simulink model "Synthgas"  (R2025a)
settings: Solver=VariableStepAuto  StartTime=0.0  StopTime=3600  RelTol=1e-3
PreLoadFcn:
  | run('params_wte.m');
  | run('PEMElectrolysisSystemParameters.m');
  | run('params_co2el.m');
InitFcn:
  | run(fullfile(fileparts(bdroot),'params_wte.m'));
  | run(fullfile(fileparts(bdroot),'PEMElectrolysisSystemParameters.m'));
  | run(fullfile(fileparts(bdroot),'params_co2el.m'));
values from neighbouring files (symbols this model uses):
  A = [ -1/tauQ,        0 ... (first row only)    [params_wte.m]
  A_cm2 = 200    [params_co2el.m]
  alpha = wC * eta_burn * (44/12)    (= 1.43733333333)    [params_wte.m]
  B = [ (eta_th*LHV)/(1e6*tauQ) ... (first row only)    [params_wte.m]
  C = [0, 1]    [params_wte.m]
  D = 0    [params_wte.m]
  env_T = 20    [PEMElectrolysisSystemParameters.m]
  exchanger_air_area_fins = 2 * exchanger_N_fins * exchanger_W * exchanger_gap_H    (= 11.5625)    [PEMElectrolysisSystemParameters.m]
  exchanger_air_area_primary = 2 * (exchanger_N_tubes - 1) * exchanger_W * (exchanger_L + exchanger_gap_H)    (= 1.223125)    [PEMElectrolysisSystemParameters.m]
  exchanger_eta_fin = 0.7    [PEMElectrolysisSystemParameters.m]
  exchanger_N_tubes = 25    [PEMElectrolysisSystemParameters.m]
  exchanger_tube_H = 0.0015    [PEMElectrolysisSystemParameters.m]
  exchanger_W = 0.025    [PEMElectrolysisSystemParameters.m]
  F = 96485.33212    [params_co2el.m]
  gas_pipe_D = 0.01    [PEMElectrolysisSystemParameters.m]
  j_tab_mAcm2 = [0 ... (first row only)    [params_co2el.m]
  MW_CO = 28.0101e-3    (= 0.0280101)    [params_co2el.m]
  MW_CO2 = 44.0095e-3    (= 0.0440095)    [params_co2el.m]
  MW_H2 = 2.01588e-3    (= 0.00201588)    [params_co2el.m]
  N2_T = [-56.55, -50:10:-10, -5:1:5, 10:10:350]    [PEMElectrolysisSystemParameters.m]
  N_cell = 200    [params_co2el.m]
  p_bp = [0 ... (first row only)    [params_co2el.m]
  P_stack_max_W = p_max * (N_cell*A_cm2) / 1000    [params_co2el.m]
  stack_area = 280    [PEMElectrolysisSystemParameters.m]
  stack_mea_rho = 1800    [PEMElectrolysisSystemParameters.m]
  stack_num_cells = 50    [PEMElectrolysisSystemParameters.m]
  stack_num_channels = 8    [PEMElectrolysisSystemParameters.m]
  stack_t_gdl_A = 25    [PEMElectrolysisSystemParameters.m]
  stack_t_gdl_C = 250    [PEMElectrolysisSystemParameters.m]
  stack_t_membrane = 125    [PEMElectrolysisSystemParameters.m]
  stack_w_channels = 1    [PEMElectrolysisSystemParameters.m]
  V_tab = [0 ... (first row only)    [params_co2el.m]
  water_pipe_D = 0.01    [PEMElectrolysisSystemParameters.m]
undefined symbols (not defined in the file or in its folder): H2O, O2
libraries: fl_lib x48, nesl_utility x12, slpidlib x3
(part 1 of 3)
settings Model: Creator=ALW  LastModifiedBy=ALW

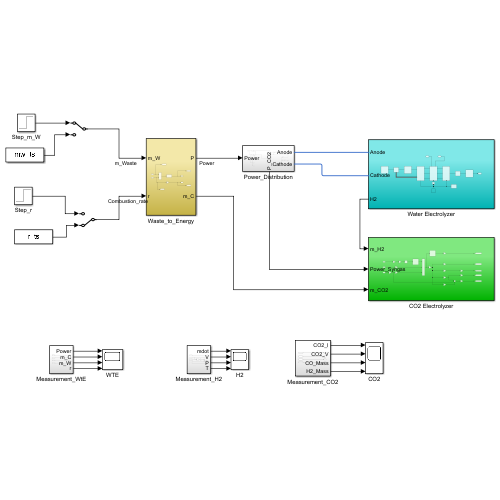
[thumbnail: Simulink's stored preview of the top-level diagram]
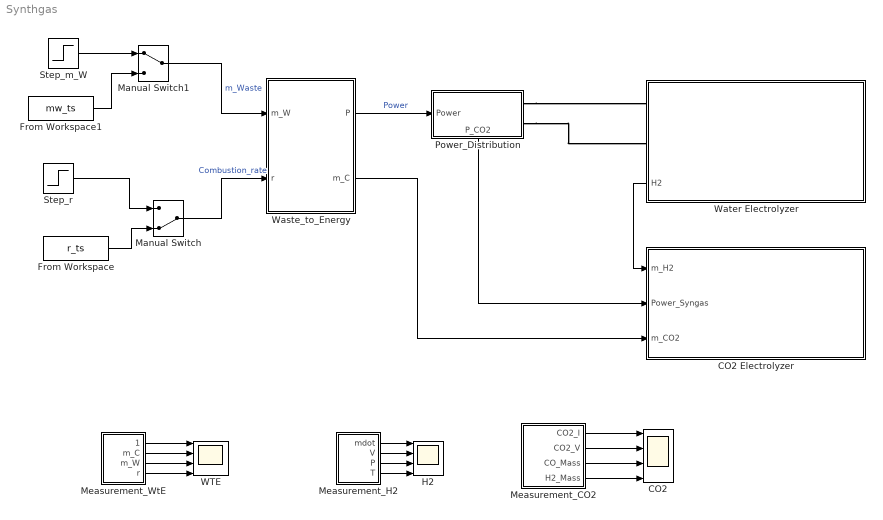
== system Synthgas ==
  CO2 : Scope  NumInputPorts=4
      settings: ActiveDisplayString=4  Title=H2 Mass Flow (g/s)  ActiveDisplayYMinimum=-0.030857277334398751  ActiveDisplayYMaximum=0.17485652421311373  DataLoggingVariableName=ScopeData2
  CO2 Electrolyzer : Subsystem
  From Workspace : FromWorkspace  VariableName=r_ts
  From Workspace1 : FromWorkspace  VariableName=mw_ts  SampleTime=-1
  H2 : Scope  NumInputPorts=4
      settings: TimeUnits=Metric (based on Time Span)  Title=Voltage (V)  ActiveDisplayYMinimum=53.882228032448204  ActiveDisplayYMaximum=104.10341408739258
  Manual Switch : ManualSwitch  CurrentSetting=0
  Manual Switch1 : ManualSwitch
  Measurement_CO2 : Subsystem
  Measurement_H2 : Subsystem
  Measurement_WtE : Subsystem
  Power_Distribution : Subsystem
      settings: PortSchema="{\"entries\":[{\"content\":{\"sides\":[{\"content\":{\"connectorIds\":[\"In1\"]},\"type\":\"ConnectorPlacement.EquallySpacedRectSide\",\"uuid\":\"a5e91349-f433-411d-b9f8-621e501842af\"},{\"content\":{\"connectorIds\":[\"RConn1\",\"RConn2\"],\"side\":\"RIGHT\"},\"type\":\"ConnectorPlacement.EquallySpacedRectSide\",\"uuid\":\"bac18b84-652b-4e68-8662-e19dcfd0b82e\"},{\"content\":{\"side\":\"TOP\"},\"type\":\"ConnectorPlacement.EquallySpacedRectSide\",\"uuid\":\"f0b6a344-7a45-434f-be8b-12a1003c411a\"},{\"content\":{\"connectorIds\":[\"Out1\"],\"side\":\"BOTTOM\"},\"type\":\"ConnectorPlacement.EquallySpacedRectSide\",\"uuid\":\"396825fb-ddc9-409b-9a7c-77fdc98f1d9d\"}]},\"type\":\"ConnectorPlacement.EquallySpacedConnector\",\"uuid\":\"de2e4aa6-0d93-42dc-b86d-8f915b9cbcf8\"}],\"packageUris\":[\"http://schema.mathworks.com/mf0/Connector/R2020b\"],\"version\":\"1.0\"}"
  Step_m_W : Step  After=0.45  SampleTime=0
  Step_r : Step  SampleTime=0
  WTE : Scope  NumInputPorts=4
      settings: ActiveDisplayString=4  Title=Combustion Rate  ActiveDisplayYMinimum=0.54999999999999993  ActiveDisplayYMaximum=1.05
  Waste_to_Energy : Subsystem
  Water Electrolyzer : Subsystem
      settings: PortSchema="{\"entries\":[{\"content\":{\"sides\":[{\"content\":{\"connectorIds\":[\"LConn1\",\"LConn2\",\"Out1\"]},\"type\":\"ConnectorPlacement.EquallySpacedRectSide\",\"uuid\":\"8c825195-5e57-4450-b541-7bc6f9239a39\"},{\"content\":{\"side\":\"RIGHT\"},\"type\":\"ConnectorPlacement.EquallySpacedRectSide\",\"uuid\":\"b534c7d2-21ee-4996-8839-3ecdb349ca3b\"},{\"content\":{\"side\":\"TOP\"},\"type\":\"ConnectorPlacement.EquallySpacedRectSide\",\"uuid\":\"d8abb2df-546c-43c5-acd7-e7d66907377d\"}]},\"type\":\"ConnectorPlacement.EquallySpacedConnector\",\"uuid\":\"cb332e70-8d84-49b3-af99-40c603273fe2\"}],\"packageUris\":[\"http://schema.mathworks.com/mf0/Connector/R2020b\"],\"version\":\"1.0\"}"
  wires:
  Step_r/1 -> Manual Switch/1
  Waste_to_Energy/1(P) -> Power_Distribution/1(Power)  "Power"
  From Workspace/1 -> Manual Switch/2
  Manual Switch/1 -> Waste_to_Energy/2(r)  "Combustion_rate"
  Step_m_W/1 -> Manual Switch1/1
  From Workspace1/1 -> Manual Switch1/2
  Manual Switch1/1 -> Waste_to_Energy/1(m_W)  "m_Waste"
  Measurement_H2/2(V) -> H2/2
  Measurement_H2/1(mdot) -> H2/1
  Measurement_H2/3(P) -> H2/3
  Measurement_H2/4(T) -> H2/4
  Measurement_WtE/1(Power) -> WTE/1
  Measurement_WtE/2(m_C) -> WTE/2
  Measurement_WtE/3(m_W) -> WTE/3
  Measurement_WtE/4(r) -> WTE/4
  Waste_to_Energy/2(m_C) -> CO2 Electrolyzer/3(m_CO2)
  Power_Distribution/1(P_CO2) -> CO2 Electrolyzer/2(Power_Syngas)
  Water Electrolyzer/1(H2) -> CO2 Electrolyzer/1(m_H2)
  Measurement_CO2/1(CO2_I) -> CO2/1
  Measurement_CO2/2(CO2_V) -> CO2/2
  Measurement_CO2/4(H2_Mass) -> CO2/4
  Measurement_CO2/3(CO_Mass) -> CO2/3
  connections:
  Power_Distribution/RConn1 -- Water Electrolyzer/LConn1
  Power_Distribution/RConn2 -- Water Electrolyzer/LConn2

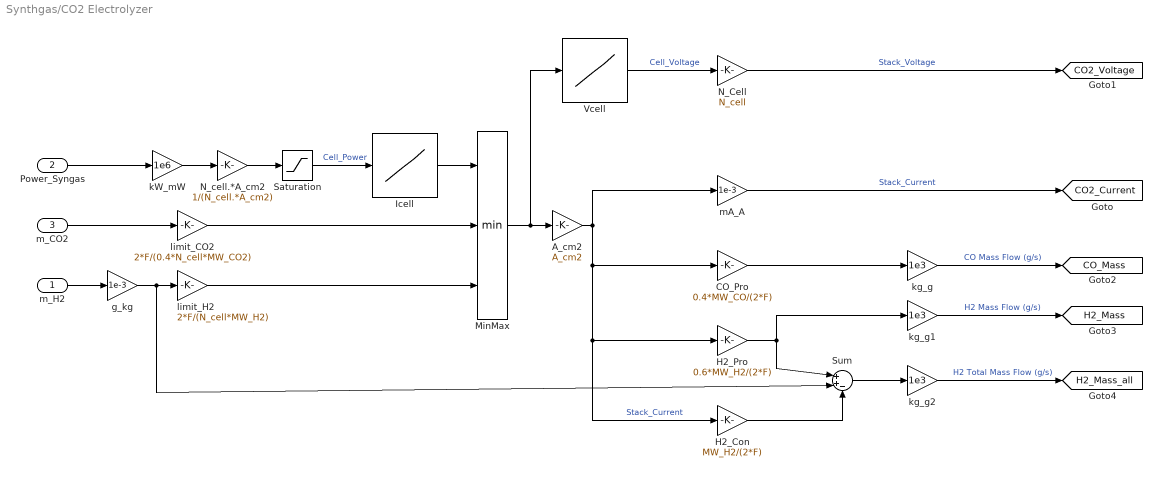
== system Synthgas/CO2 Electrolyzer ==
  m_H2 : Inport
  Power_Syngas : Inport  Port=2
  m_CO2 : Inport  Port=3
  A_cm2 : Gain  Gain=A_cm2
  CO_Pro : Gain  Gain=0.4*MW_CO/(2*F)
  H2_Con : Gain  Gain=MW_H2/(2*F)
  H2_Pro : Gain  Gain=0.6*MW_H2/(2*F)
  Icell : Lookup_n-D  NumberOfTableDimensions=1  BreakpointsForDimension1=p_bp  Table=j_tab_mAcm2  InternalRulePriority=Speed  RndMeth=Simplest
  MinMax : MinMax  Inputs=3
  N_Cell : Gain  Gain=N_cell
  N_cell.*A_cm2 : Gain  Gain=1/(N_cell.*A_cm2)
  Saturation : Saturate  UpperLimit=P_stack_max_W  LowerLimit=0
  Sum : Sum  Inputs=|++-
  Vcell : Lookup_n-D  NumberOfTableDimensions=1  BreakpointsForDimension1=j_tab_mAcm2  Table=V_tab  InternalRulePriority=Speed  RndMeth=Simplest
  g_kg : Gain  Gain=1e-3
  kW_mW : Gain  Gain=1e6
  kg_g : Gain  Gain=1e3
  kg_g1 : Gain  Gain=1e3
  kg_g2 : Gain  Gain=1e3
  limit_CO2 : Gain  Gain=2*F/(0.4*N_cell*MW_CO2)
  limit_H2 : Gain  Gain=2*F/(N_cell*MW_H2)
  mA_A : Gain  Gain=1e-3
  tag scope: CO2_Current=global, CO2_Voltage=global, CO_Mass=global, H2_Mass=global, H2_Mass_all=global
  wires:
  Sum/1 -> kg_g2/1
  A_cm2/1 -> mA_A/1, CO_Pro/1, H2_Con/1, H2_Pro/1  "Stack_Current"
  CO_Pro/1 -> kg_g/1
  N_cell.*A_cm2/1 -> Saturation/1
  H2_Pro/1 -> kg_g1/1, Sum/1
  Vcell/1 -> N_Cell/1  "Cell_Voltage"
  Saturation/1 -> Icell/1  "Cell_Power"
  N_Cell/1 -> [CO2_Voltage]  "Stack_Voltage"
  Icell/1 -> MinMax/1
  Power_Syngas/1 -> kW_mW/1
  limit_CO2/1 -> MinMax/2
  kW_mW/1 -> N_cell.*A_cm2/1
  H2_Con/1 -> Sum/3
  limit_H2/1 -> MinMax/3
  m_H2/1 -> g_kg/1
  m_CO2/1 -> limit_CO2/1
  MinMax/1 -> A_cm2/1, Vcell/1
  mA_A/1 -> [CO2_Current]  "Stack_Current"
  kg_g/1 -> [CO_Mass]  "CO Mass Flow (g/s)"
  kg_g1/1 -> [H2_Mass]  "H2 Mass Flow (g/s)"
  kg_g2/1 -> [H2_Mass_all]  "H2 Total Mass Flow (g/s)"
  g_kg/1 -> Sum/2, limit_H2/1

== system Synthgas/Measurement_CO2 ==
  CO2_I : Outport
  CO2_V : Outport  Port=2
  CO_Mass : Outport  Port=3
  H2_Mass : Outport  Port=4
  wires:
  [CO2_Current] -> CO2_I/1
  [CO2_Voltage] -> CO2_V/1
  [CO_Mass] -> CO_Mass/1
  [H2_Mass] -> H2_Mass/1

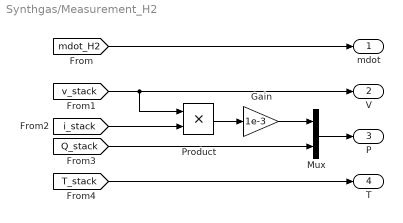
== system Synthgas/Measurement_H2 ==
  Gain : Gain  Gain=1e-3
  Mux : Mux  Inputs=2
  Product : Product
  mdot : Outport
  V : Outport  Port=2
  P : Outport  Port=3
  T : Outport  Port=4
  wires:
  [v_stack] -> Product/1, V/1
  [T_stack] -> T/1
  [Q_stack] -> Mux/2
  Product/1 -> Gain/1
  Mux/1 -> P/1
  Gain/1 -> Mux/1
  [i_stack] -> Product/2
  [mdot_H2] -> mdot/1

== system Synthgas/Measurement_WtE ==
  Power : Outport
  m_C : Outport  Port=2
  m_W : Outport  Port=3
  r : Outport  Port=4
  wires:
  [Power_WtE] -> Power/1
  [m_CO2] -> m_C/1
  [m_W] -> m_W/1
  [r] -> r/1

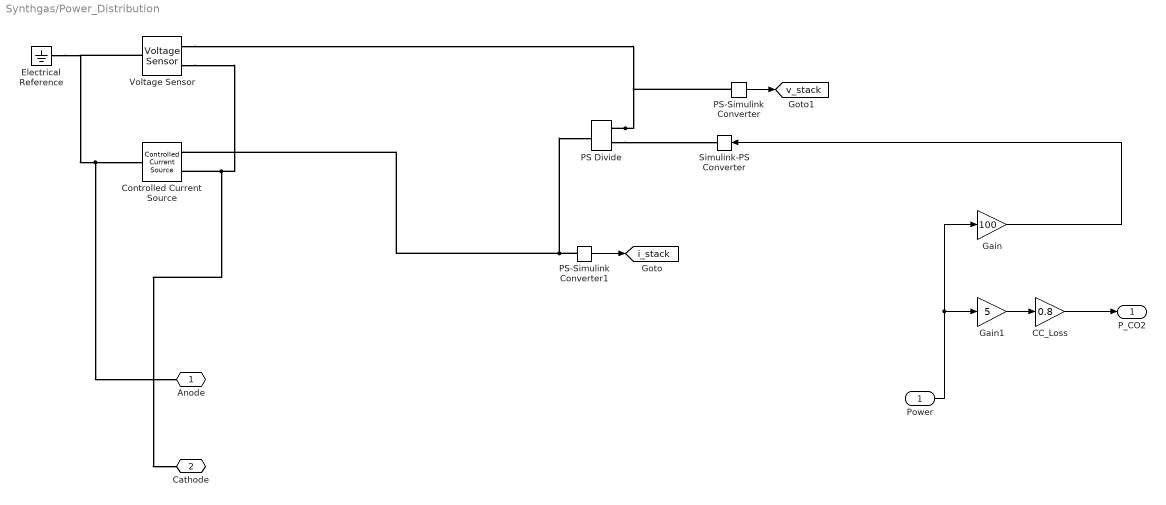
== system Synthgas/Power_Distribution ==
  Power : Inport
  CC_Loss : Gain  Gain=0.8
  Controlled Current Source : fl_lib/Electrical/Electrical Sources/Controlled Current Source
  Electrical Reference : fl_lib/Electrical/Electrical Elements/Electrical Reference
  Gain : Gain  Gain=100
  Gain1 : Gain  Gain=5
  PS Divide : fl_lib/Physical Signals/Functions/PS Divide
  PS-Simulink Converter : nesl_utility/PS-Simulink Converter  PhysicalDomain=network_engine_domain  SubClassName=ps_output  LeftPortType=input  RightPortType=output  PseudoPeriodic=off  Frequencies=[]  VectorFormat=1-D array  Unit=V  AffineConversion=off
  PS-Simulink Converter1 : nesl_utility/PS-Simulink Converter  PhysicalDomain=network_engine_domain  SubClassName=ps_output  LeftPortType=input  RightPortType=output  PseudoPeriodic=off  Frequencies=[]  VectorFormat=1-D array  Unit=A  AffineConversion=off
  Simulink-PS Converter : nesl_utility/Simulink-PS Converter  PhysicalDomain=network_engine_domain  SubClassName=ps_input  LeftPortType=input  RightPortType=output  PseudoPeriodic=off  Frequencies=[]  NoiseDistribution=none  NoiseParameters=[]  Unit=kW  AffineConversion=off  FilteringAndDerivatives=provide  SimscapeFilterOrder=1  InputFilterTimeConstant=0.001  UdotUserProvided=0
  Voltage Sensor : fl_lib/Electrical/Electrical Sensors/Voltage Sensor
  Anode : PMIOPort  Side=Right
  Cathode : PMIOPort  Port=2  Side=Right
  P_CO2 : Outport
  tag scope: i_stack=global, v_stack=global
  wires:
  PS-Simulink Converter1/1 -> [i_stack]
  PS-Simulink Converter/1 -> [v_stack]
  Power/1 -> Gain1/1, Gain/1
  Gain/1 -> Simulink-PS Converter/1
  Gain1/1 -> CC_Loss/1
  CC_Loss/1 -> P_CO2/1
  connections:
  PS Divide/LConn2 -- PS-Simulink Converter/LConn1 -- Voltage Sensor/RConn1
  Voltage Sensor/RConn2 -- Cathode/RConn1 -- Controlled Current Source/RConn2
  Electrical Reference/LConn1 -- Voltage Sensor/LConn1 -- Anode/RConn1 -- Controlled Current Source/LConn1
  PS-Simulink Converter1/LConn1 -- Controlled Current Source/RConn1 -- PS Divide/RConn1
  PS Divide/LConn1 -- Simulink-PS Converter/RConn1

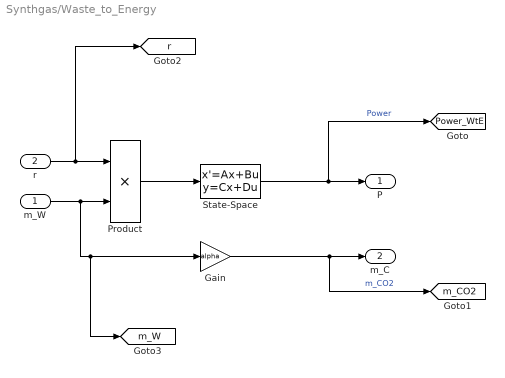
== system Synthgas/Waste_to_Energy ==
  m_W : Inport
  r : Inport  Port=2
  Gain : Gain  Gain=alpha
  Product : Product
  State-Space : StateSpace  A=A  B=B  C=C  D=D  InitialCondition=0
  P : Outport
  m_C : Outport  Port=2
  tag scope: Power_WtE=global, m_CO2=global, m_W=global, r=global
  wires:
  m_W/1 -> [m_W], Gain/1, Product/2
  State-Space/1 -> [Power_WtE], P/1  "Power"
  r/1 -> [r], Product/1
  Gain/1 -> [m_CO2], m_C/1  "m_CO2"
  Product/1 -> State-Space/1

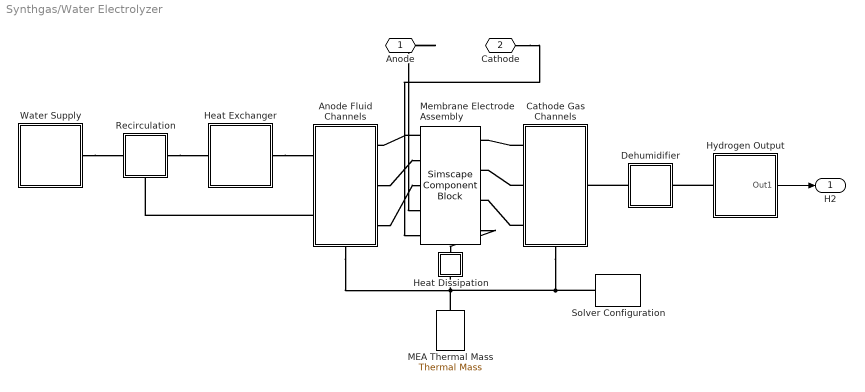
== system Synthgas/Water Electrolyzer ==
  Anode Fluid Channels : Subsystem  Tag=PublishSubsystem
      settings: PortSchema="{\"entries\":[{\"content\":{\"sides\":[{\"content\":{\"connectorIds\":[\"LConn1\",\"LConn2\"]},\"type\":\"ConnectorPlacement.EquallySpacedRectSide\",\"uuid\":\"976dc190-b3f9-4e22-888f-45b05c60a588\"},{\"content\":{\"connectorIds\":[\"RConn1\",\"RConn2\",\"RConn3\"],\"side\":\"RIGHT\"},\"type\":\"ConnectorPlacement.EquallySpacedRectSide\",\"uuid\":\"d1ee9715-6ca1-4a70-ad2c-fd039db203ea\"},{\"content\":{\"connectorIds\":[],\"side\":\"TOP\"},\"type\":\"ConnectorPlacement.EquallySpacedRectSide\",\"uuid\":\"652e2705-5c92-4089-9341-8ba766de0b19\"},{\"content\":{\"connectorIds\":[\"RConn4\"],\"side\":\"BOTTOM\"},\"type\":\"ConnectorPlacement.EquallySpacedRectSide\",\"uuid\":\"7dcfe5e1-f3b6-46fd-a931-ffa83d16832e\"}]},\"type\":\"ConnectorPlacement.EquallySpacedConnector\",\"uuid\":\"0672c964-bbe2-471b-8d85-6fb40d32f425\"}],\"packageUris\":[\"http://schema.mathworks.com/mf0/Connector/R2020b\"],\"version\":\"1.0\"}"
      mask Display:
      | plot(0, 0)
      | plot(100, 100)
      | 
      | x1 = 25;
      | x2 = 65;
      | y1 = 23;
      | y2 = 95;
      | xt = 15;
      | yt = 9;
      | 
      | x_pattern = [x2 x2    x1+xt x1+xt   x1+xt   x2     ];
      | y_pattern = [y2 y2-yt y2-yt y2-2*yt y2-2*yt y2-2*yt];
      | 
      | plot([x1 x1 x2 x_pattern x_pattern      x_pattern      x_pattern         x2    x1], ...
      |      [y1-yt y2 y2 y_pattern y_pattern-2*yt y_pattern-4*yt y_pattern-6*yt y1-yt y1-yt])
  Cathode Gas Channels : Subsystem  Tag=PublishSubsystem
      settings: PortSchema="{\"entries\":[{\"content\":{\"sides\":[{\"content\":{\"connectorIds\":[\"LConn1\",\"LConn2\",\"LConn3\"]},\"type\":\"ConnectorPlacement.EquallySpacedRectSide\",\"uuid\":\"6520ef95-25ad-4857-a8b8-cb425344d4cd\"},{\"content\":{\"connectorIds\":[\"RConn1\"],\"side\":\"RIGHT\"},\"type\":\"ConnectorPlacement.EquallySpacedRectSide\",\"uuid\":\"94443425-2825-49c6-b307-e6315f94eee5\"},{\"content\":{\"connectorIds\":[],\"side\":\"TOP\"},\"type\":\"ConnectorPlacement.EquallySpacedRectSide\",\"uuid\":\"4cac1b2b-e4ea-4d58-9811-2c1827cdae9e\"},{\"content\":{\"connectorIds\":[\"RConn2\"],\"side\":\"BOTTOM\"},\"type\":\"ConnectorPlacement.EquallySpacedRectSide\",\"uuid\":\"8cc66402-0dc1-4dc7-b90d-6a09e1b54b4f\"}]},\"type\":\"ConnectorPlacement.EquallySpacedConnector\",\"uuid\":\"a12cf322-0634-499b-9503-9d411b63f0d1\"}],\"packageUris\":[\"http://schema.mathworks.com/mf0/Connector/R2020b\"],\"version\":\"1.0\"}"
      mask Display:
      | plot(0, 0)
      | plot(100, 100)
      | 
      | x1 = 35;
      | x2 = 75;
      | y1 = 23;
      | y2 = 95;
      | xt = 15;
      | yt = 9;
      | 
      | x_pattern = [x1 x1    x2-xt x2-xt   x2-xt   x1     ];
      | y_pattern = [y2 y2-yt y2-yt y2-2*yt y2-2*yt y2-2*yt];
      | 
      | plot([x2 x2 x1 x_pattern x_pattern      x_pattern      x_pattern         x1    x2], ...
      |      [y1-yt y2 y2 y_pattern y_pattern-2*yt y_pattern-4*yt y_pattern-6*yt y1-yt y1-yt])
  Dehumidifier : Subsystem  Tag=PublishSubsystem
  Heat Dissipation : Subsystem
      settings: PortSchema="{\"entries\":[{\"content\":{\"sides\":[{\"content\":{\"connectorIds\":[]},\"type\":\"ConnectorPlacement.EquallySpacedRectSide\",\"uuid\":\"40b2385a-b20e-464f-8016-3228e4acac4a\"},{\"content\":{\"connectorIds\":[],\"side\":\"RIGHT\"},\"type\":\"ConnectorPlacement.EquallySpacedRectSide\",\"uuid\":\"0e95dc4b-d2da-4ab6-a6e9-e2cb275776ce\"},{\"content\":{\"connectorIds\":[\"LConn1\"],\"side\":\"TOP\"},\"type\":\"ConnectorPlacement.EquallySpacedRectSide\",\"uuid\":\"0f5995c7-26f6-433d-889b-dea78bcd2b2a\"},{\"content\":{\"connectorIds\":[\"RConn1\"],\"side\":\"BOTTOM\"},\"type\":\"ConnectorPlacement.EquallySpacedRectSide\",\"uuid\":\"a2ee1c19-f9e9-4dbd-a9ff-92feea387e85\"}]},\"type\":\"ConnectorPlacement.EquallySpacedConnector\",\"uuid\":\"721753ea-9ada-4c74-8c6f-50b905d96904\"}],\"packageUris\":[\"http://schema.mathworks.com/mf0/Connector/R2020b\"],\"version\":\"1.0\"}"
  Heat Exchanger : Subsystem  Tag=PublishSubsystem
      mask Display:
      | plot(0, 0)
      | plot(100, 100)
      | 
      | n = 80;
      | r = 35;
      | 
      | x = 50;
      | y = 50;
      | d = 10;
      | t = 10;
      | 
      | plot(cos(linspace(0, 2*pi, n))*r + x, sin(linspace(0, 2*pi, n))*r + y)
      | 
      | plot([0 x-r+t x-d x+d x+r-t 100], [y y y+r-t y-r+t y y])
  Hydrogen Output : Subsystem  Tag=PublishSubsystem
      mask Display:
      | plot(0, 0)
      | plot(100, 100)
      | 
      | n = 20;
      | r = 20;
      | x1 = 35;
      | x2 = 85;
      | y1 = 5;
      | y2 = 85;
      | 
      | plot([x1 x1], [y1+r y2-r])
      | plot([x1+r x2-r], [y2 y2])
      | plot([x2 x2], [y2-r y1+r])
      | plot([x2-r x1+r], [y1 y1])
      | 
      | plot(cos(linspace(pi/2, pi, n))*r + x1+r, sin(linspace(pi/2, pi, n))*r + y2-r)
      | plot(cos(linspace(0, pi/2, n))*r + x2-r, sin(linspace(0, pi/2, n))*r + y2-r)
      | plot(cos(linspace(3*pi/2, 2*pi, n))*r + x2-r, sin(linspace(3*pi/2, 2*pi, n))*r + y1+r)
      | plot(cos(linspace(pi, 3*pi/2, n))*r + x1+r, sin(linspace(pi, 3*pi/2, n))*r + y1+r)
      | 
      | plot([-5 -5 5 5] + (x1+x2)/2, [0 5 5 0] + y2)
  MEA Thermal Mass : fl_lib/Thermal/Thermal Elements/Thermal Mass  mass_type=foundation.enum.constant_variable.constant  mass=stack_mea_rho * stack_area*1e-4 * (stack_t_membrane + stack_t_gdl_A + stack_t_gdl_C)*1e-6 * stack_num_cells kg  sp_heat=stack_mea_cp J/kg/K  mass_min=1e-6 kg  num_ports=foundation.enum.numPorts2.one  m_specify=off  m_priority=High  m=1 kg  m_nominal_specify=off  m_nominal_value=1  m_nominal_unit=kg  T_specify=on  T_priority=High  T=env_T degC  T_nominal_specify=off  T_nominal_value=1  T_nominal_unit=K  Q_specify=off  Q_priority=None  Q=0 W  Q_nominal_specify=off  Q_nominal_value=1  Q_nominal_unit=W
  Membrane Electrode Assembly : SimscapeComponentBlock  SourceFile=Electrolyzer  ComponentPath=Electrolyzer  ComponentVariants="[\"Electrolyzer\"]"  ComponentVariantNames="[\"Electrolyzer\"]"  ClassName=Electrolyzer  SchemaVersion=1  N_cell=stack_num_cells  area_cell=stack_area cm^2  t_membrane=stack_t_membrane um  t_gdl_A=stack_t_gdl_A um  t_gdl_C=stack_t_gdl_C um  io=stack_io A/cm^2  alpha=stack_alpha  D_H2O_gdl_A=stack_D_gdl_A cm^2/s  D_H2O_gdl_C=stack_D_gdl_C cm^2/s  rho_membrane=stack_membrane_rho kg/m^3  M_membrane=stack_membrane_MW kg/mol  i_specify=off  i_priority=None  i=0 A  i_nominal_specify=off  i_nominal_value=1  i_nominal_unit=A  Q_specify=off  Q_priority=None  Q=0 W  Q_nominal_specify=off  Q_nominal_value=1  Q_nominal_unit=W  a_acl_specify=off  a_acl_priority=None  a_acl=0.5  a_acl_nominal_specify=off  a_acl_nominal_value=1  a_acl_nominal_unit=1  a_ccl_specify=off  a_ccl_priority=None  a_ccl=0.5  a_ccl_nominal_specify=off  a_ccl_nominal_value=1  a_ccl_nominal_unit=1  mdot_H2O_specify=off  mdot_H2O_priority=None  mdot_H2O=0 kg/s  mdot_H2O_nominal_specify=off  mdot_H2O_nominal_value=1  mdot_H2O_nominal_unit=kg/s  Phi_H2O_specify=off  Phi_H2O_priority=None  Phi_H2O=0 kW  Phi_H2O_nominal_specify=off  Phi_H2O_nominal_value=1  Phi_H2O_nominal_unit=kW
      settings: CopyFcn=simscape.sscblock.internal.componentBlockCallback(gcbh,'COPY')  PreCopyFcn=simscape.sscblock.internal.componentBlockCallback(gcbh,'PRECOPY')  PreDeleteFcn=simscape.sscblock.internal.componentBlockCallback(gcbh,'PREDELETE')  InternalSimscapePortConfiguration="{\"Bottom\":[{\"id\":\"H\",\"label\":\"H\",\"type\":\"foundation.thermal.thermal\"}],\"Left\":[{\"id\":\"A\",\"label\":\"A\",\"type\":\"foundation.moist_air.moist_air\"},{\"id\":\"H2O\",\"label\":\"H2O\",\"type\":\"foundation.thermal_liquid.thermal_liquid\"},{\"id\":\"O2\",\"label\":\"O2\",\"type\":\"foundation.moist_air.moist_air_source\"}],\"Right\":[{\"id\":\"C\",\"label\":\"C\",\"type\":\"foundation.moist_air.moist_air\"},{\"id\":\"H2\",\"label\":\"H2\",\"type\":\"foundation.moist_air.moist_air_source\"},{\"id\":\"FC\",\"label\":\"FC\",\"type\":\"input\"}],\"Top\":[{\"id\":\"p\",\"label\":\"+\",\"type\":\"foundation.electrical.electrical\"},{\"id\":\"n\",\"label\":\"-\",\"type\":\"foundation.electrical.electrical\"}]}"
      mask Type: Electrolyzer
  Recirculation : Subsystem  Tag=PublishSubsystem
      settings: PortSchema="{\"entries\":[{\"content\":{\"sides\":[{\"content\":{\"connectorIds\":[\"LConn1\"]},\"type\":\"ConnectorPlacement.EquallySpacedRectSide\",\"uuid\":\"c47f9660-fc18-4f23-8cbf-f692f8fde64e\"},{\"content\":{\"connectorIds\":[\"RConn1\"],\"side\":\"RIGHT\"},\"type\":\"ConnectorPlacement.EquallySpacedRectSide\",\"uuid\":\"c2614b4a-af33-4a10-b49b-c89e1764e644\"},{\"content\":{\"connectorIds\":[],\"side\":\"TOP\"},\"type\":\"ConnectorPlacement.EquallySpacedRectSide\",\"uuid\":\"e37e301f-fa6a-4e6c-985e-f7b15098b2f5\"},{\"content\":{\"connectorIds\":[\"RConn2\"],\"side\":\"BOTTOM\"},\"type\":\"ConnectorPlacement.EquallySpacedRectSide\",\"uuid\":\"366101c1-7068-4632-8c99-08eb58fcadd6\"}]},\"type\":\"ConnectorPlacement.EquallySpacedConnector\",\"uuid\":\"e26e63cc-dc3e-4de6-a4bb-9b3faa73a99e\"}],\"packageUris\":[\"http://schema.mathworks.com/mf0/Connector/R2020b\"],\"version\":\"1.0\"}"
  Solver Configuration : nesl_utility/Solver Configuration  PhysicalDomain=network_engine_domain  SubClassName=solver  LeftPortType=input  RightPortType=generic  Tones=[]  Harmonics=[]  SimulateNoise=off  Profile=off  UseLocalSampling=off  EnableSwitchedLinearOptims=on  FrequencyDomain=off  UseCCode=off  RelTol=0.001  AbsTol=0.001  MinStep=1e-09  ToWorkspace=off  RevertToSquareIcSolve=off  NumHomotopyIterations=100  PhasorMode=off  PhasorModeNumHarmonics=1  ConsistencySolver=NEWTON_XTOL_AFTER_FTOL  IndexReductionMethod=DerivativeReplacement  DoDC=off  ResidualTolerance=1e-09  ConsistencyTolSource=GLOBAL  ConsistencyAbsTol=0.001  ConsistencyRelTol=0.001  ConsistencyTolFactor=0.001  UseLocalSolver=off  LocalSolverChoice=NE_BACKWARD_EULER_ADVANCER  ResolveIndetEquations=on  FunctionEvalNumThread=1  LocalSolverSampleTime=0.001  DoFixedCost=off  MaxNonlinIter=3  MaxModeIter=2  ComputeImpulses=off  ImpulseIterations=2  LinearAlgebra=auto  LinearAlgebraNumThread=0  EquationFormulation=NE_TIME_EF  DelaysMemoryBudget=1024  AutomaticFiltering=on  FilteringTimeConstant=0.001  PartitionStorageMethod=AS_NEEDED  PartitionMemoryBudget=1024  PartitionMethod=ROBUST  MultibodyUseLocalSolver=off  MultibodyLocalSolverChoice=ODE1  MultibodyLocalSolverSampleTime=0.001
  Water Supply : Subsystem  Tag=PublishSubsystem
      mask Display:
      | plot(0, 0)
      | plot(100, 100)
      | 
      | x = 35;
      | y = 50;
      | w = 25;
      | h = 35;
      | t = 5;
      | 
      | plot([x-w-t x-w x-w x+w x+w x+w+t], [y+h y+h y-h y-h y+h y+h])
      | plot([x-w x+w], [60 60])
      | plot([x x+t]-15, [y y]-10)
      | plot([x x+t]+8, [y y]+0)
      | plot([x x+t]+12, [y y]-25)
      | plot([x x+t]-5, [y y]-20)
  Anode : PMIOPort  Side=Left
  Cathode : PMIOPort  Port=2  Side=Left
  H2 : Outport
  wires:
  Hydrogen Output/1(Out1) -> H2/1
  connections:
  Anode Fluid Channels/RConn3 -- Membrane Electrode Assembly/LConn3
  Membrane Electrode Assembly/LConn1 -- Anode Fluid Channels/RConn1
  Membrane Electrode Assembly/RConn4 -- Heat Dissipation/LConn1
  Cathode Gas Channels/LConn1 -- Membrane Electrode Assembly/RConn1
  Recirculation/RConn1 -- Heat Exchanger/LConn1
  Hydrogen Output/LConn1 -- Dehumidifier/RConn1
  Anode Fluid Channels/LConn2 -- Recirculation/RConn2
  Anode/RConn1 -- Membrane Electrode Assembly/LConn4
  Water Supply/RConn1 -- Recirculation/LConn1
  Cathode Gas Channels/LConn3 -- Membrane Electrode Assembly/RConn3
  Solver Configuration/RConn1 -- Anode Fluid Channels/RConn4 -- Heat Dissipation/RConn1 -- MEA Thermal Mass/LConn1 -- Cathode Gas Channels/RConn2
  Anode Fluid Channels/RConn2 -- Membrane Electrode Assembly/LConn2
  Cathode Gas Channels/LConn2 -- Membrane Electrode Assembly/RConn2
  Dehumidifier/LConn1 -- Cathode Gas Channels/RConn1
  Heat Exchanger/RConn1 -- Anode Fluid Channels/LConn1
  Cathode/RConn1 -- Membrane Electrode Assembly/LConn5

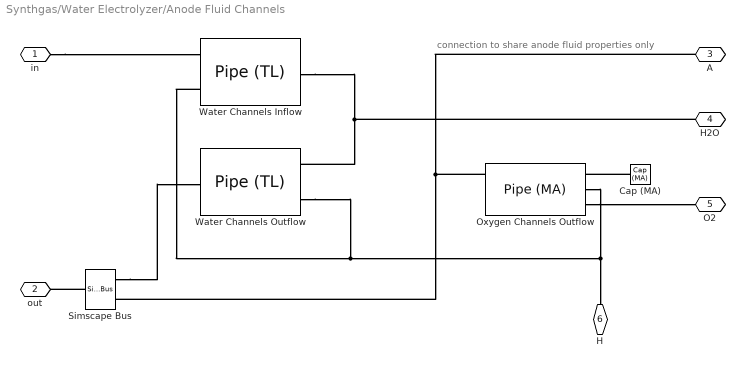
== system Synthgas/Water Electrolyzer/Anode Fluid Channels ==
  note: connection to share anode fluid properties only
  Cap (MA) : fl_lib/Moist Air/Elements/Cap (MA)  p_specify=off  p_priority=None  p=0.1 MPa  p_nominal_specify=off  p_nominal_value=1  p_nominal_unit=MPa  T_specify=off  T_priority=None  T=300 K  T_nominal_specify=off  T_nominal_value=1  T_nominal_unit=K  x_w_specify=off  x_w_priority=None  x_w=0  x_w_nominal_specify=off  x_w_nominal_value=1  x_w_nominal_unit=1  x_g_specify=off  x_g_priority=None  x_g=0  x_g_nominal_specify=off  x_g_nominal_value=1  x_g_nominal_unit=1  r_d_specify=off  r_d_priority=None  r_d=0  r_d_nominal_specify=off  r_d_nominal_value=1  r_d_nominal_unit=1
      settings: InternalSimscapePortConfiguration="{\"Bottom\":[],\"Left\":[{\"id\":\"A\",\"label\":\"\",\"type\":\"foundation.moist_air.moist_air\"}],\"Right\":[],\"Top\":[]}"
  Oxygen Channels Outflow : fl_lib/Moist Air/Elements/Pipe (MA)  length=sqrt(stack_area) cm  area=stack_w_channels^2 * stack_num_channels * stack_num_cells cm^2  Dh=stack_w_channels cm  length_add=1 m  roughness=15e-6 m  Re_lam=2000  Re_tur=4000  shape_factor=64  Nu_lam=3.66  wall_condensation=simscape.enum.onoff.off  RH_ws=1  time_constant_cond=1e-3 s  time_constant_evap=1e-3 s  fraction_entrained=1  moisture_trace_gas_source=foundation.enum.moisture_trace_gas_source.controlled  moisture_source_spec=foundation.enum.MoistureSourceSpec.WaterVapor  vapor_from_liquid=false  moisture_mass_flow=0 kg/s  moisture_temperature_spec=foundation.enum.temperature_spec.atmospheric  moisture_temperature=293.15 K  trace_gas_mass_flow=0 kg/s  trace_gas_temperature_spec=foundation.enum.temperature_spec.atmospheric  trace_gas_temperature=293.15 K  p_init=env_p MPa  p_init_priority=foundation.enum.Priority.High  T_init=env_T degC  T_init_priority=foundation.enum.Priority.High  humidity_spec=foundation.enum.HumiditySpec.MoleFraction  RH_init=0  RH_init_priority=foundation.enum.Priority.None  x_w_init=0  x_w_init_priority=foundation.enum.Priority.None  y_w_init=0  y_w_init_priority=foundation.enum.Priority.High  HR_init=0  HR_init_priority=foundation.enum.Priority.None  Tw_init=287 K  Tw_init_priority=foundation.enum.Priority.High  trace_gas_spec=foundation.enum.trace_gas_spec.mole_fraction  x_g_init=1  x_g_init_priority=foundation.enum.Priority.None  y_g_init=1  y_g_init_priority=foundation.enum.Priority.High  r_d_init=0  r_d_init_priority=foundation.enum.Priority.High
      settings: InternalSimscapePortConfiguration="{\"Bottom\":[],\"Left\":[{\"id\":\"A\",\"label\":\"A\",\"type\":\"foundation.moist_air.moist_air\"},{\"id\":\"H\",\"label\":\"H\",\"type\":\"foundation.thermal.thermal\"},{\"id\":\"S\",\"label\":\"S\",\"type\":\"foundation.moist_air.moist_air_source\"}],\"Right\":[{\"id\":\"B\",\"label\":\"B\",\"type\":\"foundation.moist_air.moist_air\"},{\"id\":\"W\",\"label\":\"W\",\"type\":\"output\"},{\"id\":\"F\",\"label\":\"F\",\"type\":\"output\"}],\"Top\":[]}"
  Simscape Bus : SimscapeBus  HierarchyStrings=H2O;O2
  Water Channels Inflow : fl_lib/Thermal Liquid/Elements/Pipe (TL)  length=sqrt(stack_area) / 2 cm  area=stack_w_channels^2 * stack_num_channels * stack_num_cells cm^2  Dh=stack_w_channels cm  length_add=1 cm  roughness=15e-6 m  Re_lam=2000  Re_tur=4000  shape_factor=64  Nu_lam=3.66  dynamic_compressibility=simscape.enum.onoff.on  inertia=simscape.enum.onoff.off  p0=env_p MPa  T0=env_T degC  mdot0=0 kg/s  p_nominal=0.101325 MPa  T_nominal=293.15 K
  Water Channels Outflow : fl_lib/Thermal Liquid/Elements/Pipe (TL)  length=sqrt(stack_area) / 2 cm  area=stack_w_channels^2 * stack_num_channels * stack_num_cells cm^2  Dh=stack_w_channels cm  length_add=1 cm  roughness=15e-6 m  Re_lam=2000  Re_tur=4000  shape_factor=64  Nu_lam=3.66  dynamic_compressibility=simscape.enum.onoff.on  inertia=simscape.enum.onoff.off  p0=env_p MPa  T0=env_T degC  mdot0=0 kg/s  p_nominal=0.101325 MPa  T_nominal=293.15 K
  in : PMIOPort  Side=Left
  out : PMIOPort  Port=2  Side=Left
  A : PMIOPort  Port=3  Side=Right
  H2O : PMIOPort  Port=4  Side=Right
  O2 : PMIOPort  Port=5  Side=Right
  H : PMIOPort  Port=6  Side=Right
  connections:
  in/RConn1 -- Water Channels Inflow/LConn1
  Water Channels Inflow/RConn1 -- Water Channels Outflow/LConn1 -- H2O/RConn1
  Water Channels Inflow/LConn2 -- H/RConn1 -- Oxygen Channels Outflow/LConn2 -- Water Channels Outflow/LConn2
  Oxygen Channels Outflow/RConn1 -- Simscape Bus/LConn2 -- A/RConn1
  Simscape Bus/LConn1 -- Water Channels Outflow/RConn1
  Simscape Bus/RConn1 -- out/RConn1
  Oxygen Channels Outflow/LConn3 -- O2/RConn1
  Cap (MA)/LConn1 -- Oxygen Channels Outflow/LConn1

== system Synthgas/Water Electrolyzer/Cathode Gas Channels ==
  note: connection to share cathode fluid properties only
  Cap (MA) : fl_lib/Moist Air/Elements/Cap (MA)  p_specify=off  p_priority=None  p=0.1 MPa  p_nominal_specify=off  p_nominal_value=1  p_nominal_unit=MPa  T_specify=off  T_priority=None  T=300 K  T_nominal_specify=off  T_nominal_value=1  T_nominal_unit=K  x_w_specify=off  x_w_priority=None  x_w=0  x_w_nominal_specify=off  x_w_nominal_value=1  x_w_nominal_unit=1  x_g_specify=off  x_g_priority=None  x_g=0  x_g_nominal_specify=off  x_g_nominal_value=1  x_g_nominal_unit=1  r_d_specify=off  r_d_priority=None  r_d=0  r_d_nominal_specify=off  r_d_nominal_value=1  r_d_nominal_unit=1
      settings: InternalSimscapePortConfiguration="{\"Bottom\":[],\"Left\":[{\"id\":\"A\",\"label\":\"\",\"type\":\"foundation.moist_air.moist_air\"}],\"Right\":[],\"Top\":[]}"
  Hydrogen Channels Outflow : fl_lib/Moist Air/Elements/Pipe (MA)  length=sqrt(stack_area) cm  area=stack_w_channels^2 * stack_num_channels * stack_num_cells cm^2  Dh=stack_w_channels cm  length_add=1 cm  roughness=15e-6 m  Re_lam=2000  Re_tur=4000  shape_factor=64  Nu_lam=3.66  wall_condensation=simscape.enum.onoff.off  RH_ws=1  time_constant_cond=1e-3 s  time_constant_evap=1e-3 s  fraction_entrained=1  moisture_trace_gas_source=foundation.enum.moisture_trace_gas_source.controlled  moisture_source_spec=foundation.enum.MoistureSourceSpec.WaterVapor  vapor_from_liquid=false  moisture_mass_flow=0 kg/s  moisture_temperature_spec=foundation.enum.temperature_spec.atmospheric  moisture_temperature=293.15 K  trace_gas_mass_flow=0 kg/s  trace_gas_temperature_spec=foundation.enum.temperature_spec.atmospheric  trace_gas_temperature=293.15 K  p_init=env_p MPa  p_init_priority=foundation.enum.Priority.High  T_init=env_T degC  T_init_priority=foundation.enum.Priority.High  humidity_spec=foundation.enum.HumiditySpec.MoleFraction  RH_init=0  RH_init_priority=foundation.enum.Priority.None  x_w_init=0  x_w_init_priority=foundation.enum.Priority.None  y_w_init=0  y_w_init_priority=foundation.enum.Priority.High  HR_init=0  HR_init_priority=foundation.enum.Priority.None  Tw_init=287 K  Tw_init_priority=foundation.enum.Priority.High  trace_gas_spec=foundation.enum.trace_gas_spec.mole_fraction  x_g_init=1  x_g_init_priority=foundation.enum.Priority.None  y_g_init=1  y_g_init_priority=foundation.enum.Priority.High  r_d_init=0  r_d_init_priority=foundation.enum.Priority.High
      settings: InternalSimscapePortConfiguration="{\"Bottom\":[],\"Left\":[{\"id\":\"A\",\"label\":\"A\",\"type\":\"foundation.moist_air.moist_air\"},{\"id\":\"H\",\"label\":\"H\",\"type\":\"foundation.thermal.thermal\"},{\"id\":\"S\",\"label\":\"S\",\"type\":\"foundation.moist_air.moist_air_source\"}],\"Right\":[{\"id\":\"B\",\"label\":\"B\",\"type\":\"foundation.moist_air.moist_air\"},{\"id\":\"W\",\"label\":\"W\",\"type\":\"output\"},{\"id\":\"F\",\"label\":\"F\",\"type\":\"output\"}],\"Top\":[]}"
  C : PMIOPort  Side=Left
  H2 : PMIOPort  Port=2  Side=Left
  FC : PMIOPort  Port=3  Side=Left
  out : PMIOPort  Port=4  Side=Right
  H : PMIOPort  Port=5  Side=Right
  connections:
  out/RConn1 -- Hydrogen Channels Outflow/RConn1 -- C/RConn1
  H/RConn1 -- Hydrogen Channels Outflow/LConn2
  Hydrogen Channels Outflow/LConn3 -- H2/RConn1
  Hydrogen Channels Outflow/RConn3 -- FC/RConn1
  Cap (MA)/LConn1 -- Hydrogen Channels Outflow/LConn1

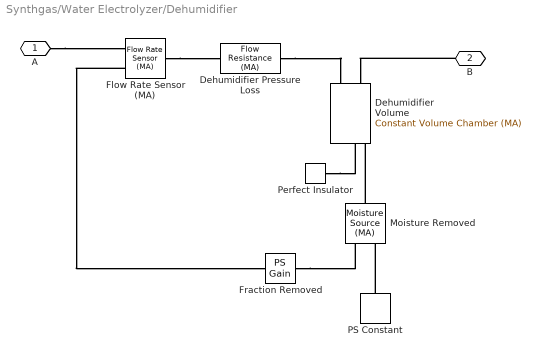
== system Synthgas/Water Electrolyzer/Dehumidifier ==
  Dehumidifier Pressure Loss : fl_lib/Moist Air/Elements/Flow Resistance (MA)  delta_p_nominal=0.001 MPa  mdot_nominal=1e-3 kg/s  rho_nominal=0.18 kg/m^3  area=pi*gas_pipe_D^2/4 m^2  laminar_fraction=1e-3
  Dehumidifier Volume : fl_lib/Moist Air/Elements/Constant Volume Chamber (MA)  volume=1e-4 m^3  num_ports=foundation.enum.num_ports.two  area_A=pi*gas_pipe_D^2/4 m^2  area_B=pi*gas_pipe_D^2/4 m^2  area_C=0.01 m^2  area_D=0.01 m^2  RH_ws=1  time_constant_cond=1e-3 s  time_constant_evap=1e-3 s  fraction_entrained=1  moisture_trace_gas_source=foundation.enum.moisture_trace_gas_source.controlled  moisture_source_spec=foundation.enum.MoistureSourceSpec.WaterVapor  vapor_from_liquid=false  moisture_mass_flow=0 kg/s  moisture_temperature_spec=foundation.enum.temperature_spec.atmospheric  moisture_temperature=293.15 K  trace_gas_mass_flow=0 kg/s  trace_gas_temperature_spec=foundation.enum.temperature_spec.atmospheric  trace_gas_temperature=293.15 K  p_init=env_p MPa  p_init_priority=foundation.enum.Priority.High  T_init=env_T degC  T_init_priority=foundation.enum.Priority.High  humidity_spec=foundation.enum.HumiditySpec.MoleFraction  RH_init=0  RH_init_priority=foundation.enum.Priority.None  x_w_init=0  x_w_init_priority=foundation.enum.Priority.None  y_w_init=1e-6  y_w_init_priority=foundation.enum.Priority.High  HR_init=0  HR_init_priority=foundation.enum.Priority.None  Tw_init=287 K  Tw_init_priority=foundation.enum.Priority.High  trace_gas_spec=foundation.enum.trace_gas_spec.mole_fraction  x_g_init=1  x_g_init_priority=foundation.enum.Priority.None  y_g_init=1 - 2e-6  y_g_init_priority=foundation.enum.Priority.High  r_d_init=0  r_d_init_priority=foundation.enum.Priority.High
      settings: InternalSimscapePortConfiguration="{\"Bottom\":[],\"Left\":[{\"id\":\"A\",\"label\":\"A\",\"type\":\"foundation.moist_air.moist_air\"},{\"id\":\"B\",\"label\":\"B\",\"type\":\"foundation.moist_air.moist_air\"}],\"Right\":[{\"id\":\"W\",\"label\":\"W\",\"type\":\"output\"},{\"id\":\"F\",\"label\":\"F\",\"type\":\"output\"},{\"id\":\"H\",\"label\":\"H\",\"type\":\"foundation.thermal.thermal\"},{\"id\":\"S\",\"label\":\"S\",\"type\":\"foundation.moist_air.moist_air_source\"}],\"Top\":[]}"
  Flow Rate Sensor (MA) : fl_lib/Moist Air/Sensors/Flow Rate Sensor (MA)  mass_flow_measure=false  volumetric_flow_measure=false  volumetric_flow_conditions=foundation.enum.volumetric_flow_conditions.actual  p_std=0.101325 MPa  T_std=20 degC  RH_std=0.65  energy_flow_measure=false  vapor_flow_measure=true  gas_flow_measure=false  droplets_flow_measure=false
      settings: InternalSimscapePortConfiguration="{\"Bottom\":[],\"Left\":[{\"id\":\"A\",\"label\":\"A\",\"type\":\"foundation.moist_air.moist_air\"},{\"id\":\"Mw\",\"label\":\"Mw\",\"type\":\"output\"}],\"Right\":[{\"id\":\"B\",\"label\":\"B\",\"type\":\"foundation.moist_air.moist_air\"}],\"Top\":[]}"
  Fraction Removed : fl_lib/Physical Signals/Functions/PS Gain  gain=-0.999
  Moisture Removed : fl_lib/Moist Air/Sources/Moisture & Trace Gas Sources/Moisture Source (MA)  source_type=foundation.enum.constant_controlled.controlled  moisture_source_spec=foundation.enum.MoistureSourceSpec.WaterVapor  vapor_from_liquid=false  moisture_mass_flow=0 kg/s  temperature_spec=foundation.enum.temperature_spec.atmospheric  moisture_temperature=293.15 K  Phi_S_specify=off  Phi_S_priority=None  Phi_S=0 kW  Phi_S_nominal_specify=off  Phi_S_nominal_value=1  Phi_S_nominal_unit=kW  mdot_w_S_specify=off  mdot_w_S_priority=None  mdot_w_S=0 kg/s  mdot_w_S_nominal_specify=off  mdot_w_S_nominal_value=1  mdot_w_S_nominal_unit=kg/s  mdot_d_S_specify=off  mdot_d_S_priority=None  mdot_d_S=0 kg/s  mdot_d_S_nominal_specify=off  mdot_d_S_nominal_value=1  mdot_d_S_nominal_unit=kg/s
      settings: InternalSimscapePortConfiguration="{\"Bottom\":[],\"Left\":[{\"id\":\"S\",\"label\":\"S\",\"type\":\"foundation.moist_air.moist_air_source\"}],\"Right\":[{\"id\":\"M\",\"label\":\"M\",\"type\":\"input\"},{\"id\":\"T\",\"label\":\"T\",\"type\":\"input\"}],\"Top\":[]}"
  PS Constant : fl_lib/Physical Signals/Sources/PS Constant  constant=env_T + 273.15 K
  Perfect Insulator : fl_lib/Thermal/Thermal Elements/Perfect Insulator  T_specify=off  T_priority=None  T=293.15 K  T_nominal_specify=off  T_nominal_value=1  T_nominal_unit=K
  A : PMIOPort  Side=Left
  B : PMIOPort  Port=2  Side=Right
  connections:
  B/RConn1 -- Dehumidifier Volume/LConn2
  Perfect Insulator/LConn1 -- Dehumidifier Volume/RConn3
  A/RConn1 -- Flow Rate Sensor (MA)/LConn1
  Flow Rate Sensor (MA)/RConn1 -- Dehumidifier Pressure Loss/LConn1
  Moisture Removed/LConn1 -- Dehumidifier Volume/RConn4
  Flow Rate Sensor (MA)/LConn2 -- Fraction Removed/LConn1
  Fraction Removed/RConn1 -- Moisture Removed/RConn1
  PS Constant/RConn1 -- Moisture Removed/RConn2
  Dehumidifier Pressure Loss/RConn1 -- Dehumidifier Volume/LConn1

== system Synthgas/Water Electrolyzer/Heat Dissipation ==
  Heat Flow Rate Sensor : fl_lib/Thermal/Thermal Sensors/Heat Flow Rate Sensor
  PS-Simulink Converter : nesl_utility/PS-Simulink Converter  PhysicalDomain=network_engine_domain  SubClassName=ps_output  LeftPortType=input  RightPortType=output  PseudoPeriodic=off  Frequencies=[]  VectorFormat=inherit  Unit=degC  AffineConversion=on
  PS-Simulink Converter1 : nesl_utility/PS-Simulink Converter  PhysicalDomain=network_engine_domain  SubClassName=ps_output  LeftPortType=input  RightPortType=output  PseudoPeriodic=off  Frequencies=[]  VectorFormat=1-D array  Unit=kW  AffineConversion=off
  Temperature Sensor : fl_lib/Thermal/Thermal Sensors/Temperature Sensor  temperature_measure=foundation.enum.MeasurementReference.absolute
      settings: InternalSimscapePortConfiguration="{\"Bottom\":[],\"Left\":[{\"id\":\"A\",\"label\":\"A\",\"type\":\"foundation.thermal.thermal\"}],\"Right\":[{\"id\":\"T\",\"label\":\"T\",\"type\":\"output\"}],\"Top\":[]}"
  A : PMIOPort  Side=Left
  B : PMIOPort  Port=2  Side=Right
  tag scope: Q_stack=global, T_stack=global
  wires:
  PS-Simulink Converter1/1 -> [Q_stack]
  PS-Simulink Converter/1 -> [T_stack]
  connections:
  A/RConn1 -- Temperature Sensor/LConn1 -- Heat Flow Rate Sensor/LConn1
  B/RConn1 -- Heat Flow Rate Sensor/RConn2
  Heat Flow Rate Sensor/RConn1 -- PS-Simulink Converter1/LConn1
  Temperature Sensor/RConn1 -- PS-Simulink Converter/LConn1

== system Synthgas/Water Electrolyzer/Heat Exchanger ==
  Convective Heat Transfer : fl_lib/Thermal/Thermal Elements/Convective Heat Transfer  thermal_type=foundation.enum.constant_variable.constant  area=exchanger_air_area_primary + exchanger_eta_fin*exchanger_air_area_fins m^2  heat_tr_coeff=300 W/(K*m^2)  min_heat_tr_coeff=1e-3 W/(K*m^2)  T_specify=off  T_priority=None  T=0 K  T_nominal_specify=off  T_nominal_value=1  T_nominal_unit=K  Q_specify=off  Q_priority=None  Q=0 W  Q_nominal_specify=off  Q_nominal_value=1  Q_nominal_unit=W
  Environment Temperature : fl_lib/Thermal/Thermal Sources/Temperature Source  temperature=env_T degC
  Heat Exchanger : fl_lib/Thermal Liquid/Elements/Pipe (TL)  length=exchanger_L m  area=exchanger_W * exchanger_tube_H * exchanger_N_tubes m^2  Dh=2*exchanger_W*exchanger_tube_H / (exchanger_W + exchanger_tube_H) m  length_add=exchanger_tube_Leq m  roughness=15e-6 m  Re_lam=2000  Re_tur=4000  shape_factor=64  Nu_lam=3.66  dynamic_compressibility=simscape.enum.onoff.on  inertia=simscape.enum.onoff.off  p0=env_p MPa  T0=env_T degC  mdot0=0 kg/s  p_nominal=0.101325 MPa  T_nominal=293.15 K
  A : PMIOPort  Side=Left
  B : PMIOPort  Port=2  Side=Right
  connections:
  Heat Exchanger/LConn1 -- A/RConn1
  B/RConn1 -- Heat Exchanger/RConn1
  Convective Heat Transfer/RConn1 -- Heat Exchanger/LConn2
  Convective Heat Transfer/LConn1 -- Environment Temperature/LConn1
